simulink model "sampleModel2403_pp_difftest"  (R2018a)
settings: Solver=VariableStepAuto  StartTime=0.0  StopTime=10.0  RelTol=1e-3
undefined symbols (not defined in the file): DiscIntNeverNeededParam, sigbuilder_block
libraries: simulink x128
(part 1 of 3)
settings Model: Creator=cyfuzz  LastModifiedBy=ishaf
settings CodeAppCC: StateflowObjectComments=on

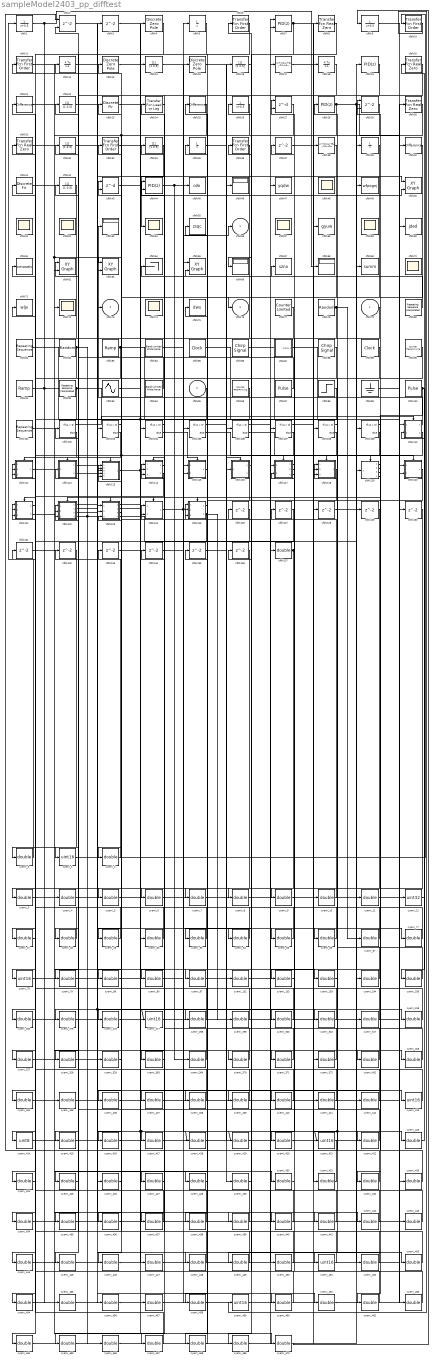
== system sampleModel2403_pp_difftest ==
  cfblk79 : Inport
  cfblk95 : Inport  Port=2
  cfblk1 : DiscreteTransferFcn  SampleTime=1
  cfblk{6,10..11,33,36} (5 alike) : simulink/Discrete/Transfer Fcn First Order  PoleZ=0.95  ICPrevOutput=0.0  DoSatur=off
      settings: SourceProductName=Simulink
  cfblk100 : DiscretePulseGenerator  PulseType=Time based  Period=10  PulseWidth=5
  cfblk101 : simulink/Sources/Repeating Sequence  rep_seq_t=[0 2]  rep_seq_y=[0 2]
  cfblk{102..109} (8 alike) : If  SampleTime=1
  cfblk110 : Subsystem  TreatAsAtomicUnit=on
  cfblk111 : Subsystem  TreatAsAtomicUnit=on
  cfblk112 : Subsystem  TreatAsAtomicUnit=on
  cfblk113 : Subsystem  TreatAsAtomicUnit=on
  cfblk114 : Subsystem  TreatAsAtomicUnit=on
  cfblk115 : Subsystem  TreatAsAtomicUnit=on
  cfblk116 : Subsystem  TreatAsAtomicUnit=on
  cfblk117 : Subsystem  TreatAsAtomicUnit=on
  cfblk118 : Subsystem  TreatAsAtomicUnit=on
  cfblk119 : Subsystem  TreatAsAtomicUnit=on
  cfblk12 : DiscreteIntegrator  OutDataTypeStr=double  ICPrevOutput=DiscIntNeverNeededParam  ICPrevScaledInput=DiscIntNeverNeededParam
  cfblk120 : Subsystem  TreatAsAtomicUnit=on
  cfblk121 : Subsystem  TreatAsAtomicUnit=on
  cfblk122 : Subsystem  TreatAsAtomicUnit=on
  cfblk123 : Subsystem  TreatAsAtomicUnit=on
  cfblk124 : Subsystem  TreatAsAtomicUnit=on
  cfblk125 : Subsystem  TreatAsAtomicUnit=on
  cfblk{3,37,126..136} (13 alike) : Delay  SampleTime=1
  cfblk13 : DiscreteZeroPole  Poles=[0 0.5]  Gain=1
  cfblk137 : DataTypeConversion  OutDataTypeStr=double
  cfblk{14,16,22,32,34,42} (6 alike) : DiscreteFilter  SampleTime=1
  cfblk15 : DiscreteZeroPole  Poles=[0 0.5]  Gain=1
  cfblk17 : DiscreteStateSpace
  cfblk18 : DiscreteIntegrator  OutDataTypeStr=double  ICPrevOutput=DiscIntNeverNeededParam  ICPrevScaledInput=DiscIntNeverNeededParam
  cfblk19 : simulink/Continuous/PID Controller  Controller=PID  TimeDomain=Discrete-time  SampleTime=1  IntegratorMethod=Forward Euler  FilterMethod=Forward Euler  Form=Parallel  UseFilter=on  ControllerParametersSource=internal  P=1  I=1  D=0  N=100  InitialConditionSource=internal  InitialConditionForIntegrator=0  InitialConditionForFilter=0  ExternalReset=none  LimitOutput=off  UpperSaturationLimit=inf  LowerSaturationLimit=-inf  LinearizeAsGain=off  AntiWindupMode=none  Kb=1  TrackingMode=off  Kt=1  PParamMin=[]  PParamMax=[]  IParamMin=[]  IParamMax=[]  DParamMin=[]  DParamMax=[]  NParamMin=[]  NParamMax=[]  KbParamMin=[]  KbParamMax=[]  KtParamMin=[]  KtParamMax=[]  POutMin=[]  POutMax=[]  IOutMin=[]  IOutMax=[]  DOutMin=[]  DOutMax=[]  NOutMin=[]  NOutMax=[]  KbOutMin=[]  KbOutMax=[]  KtOutMin=[]  KtOutMax=[]  IntegratorOutMin=[]  IntegratorOutMax=[]  FilterOutMin=[]  FilterOutMax=[]  SumOutMin=[]  SumOutMax=[]  SumI1OutMin=[]  SumI1OutMax=[]  SumI2OutMin=[]  SumI2OutMax=[]  SumI3OutMin=[]  SumI3OutMax=[]  SumDOutMin=[]  SumDOutMax=[]  SaturationOutMin=[]  SaturationOutMax=[]  IntegratorContinuousStateAttributes=''  IntegratorStateMustResolveToSignalObject=off  IntegratorRTWStateStorageClass=Auto  FilterContinuousStateAttributes=''  FilterStateMustResolveToSignalObject=off  FilterRTWStateStorageClass=Auto  DifferentiatorICPrevScaledInput=0  DifferentiatorOutMin=[]  DifferentiatorOutMax=[]  FilterDiffOutCoefMin=[]  FilterDiffOutCoefMax=[]  SumDenOutMin=[]  SumDenOutMax=[]  SumNumOutMin=[]  SumNumOutMax=[]  ReciprocalOutMin=[]  ReciprocalOutMax=[]  DivideOutMin=[]  DivideOutMax=[]  TunerSelectOption=Transfer Function Based (PID Tuner App)
  cfblk2 : Delay  ShowEnablePort=on  SampleTime=1
      settings: InputPortMap=u0,e6
  cfblk{8,20,30..31} (4 alike) : simulink/Discrete/Transfer Fcn Real Zero  ZeroZ=0.75  ICPrevInput=0.0  DoSatur=off
      settings: SourceProductName=Simulink  SourceProductBaseCode=SL
  cfblk21 : simulink/Discrete/Difference  ICPrevInput=0.0  OutMin=[]  OutMax=[]  OutDataTypeStr=double  OutputDataTypeScalingMode=double  OutDataType=fixdt(1, 16)  OutScaling=2^-10  DoSatur=off
  cfblk23 : DiscreteFir  SampleTime=1
  cfblk24 : simulink/Discrete/Transfer Fcn Lead or Lag  PoleZ=0.95  ZeroZ=0.75  ICPrevOutput=0.0  ICPrevInput=0.0  DoSatur=off
      settings: SourceProductName=Simulink  SourceProductBaseCode=SL
  cfblk25 : simulink/Discrete/Difference  ICPrevInput=0.0  OutMin=[]  OutMax=[]  OutDataTypeStr=double  OutputDataTypeScalingMode=double  OutDataType=fixdt(1, 16)  OutScaling=2^-10  DoSatur=off
  cfblk26 : DiscreteTransferFcn  SampleTime=1
  cfblk27 : Delay  DelayLengthSource=Input port  SampleTime=1
      settings: InputPortMap=u0,p1
  cfblk28 : simulink/Continuous/PID Controller  Controller=PID  TimeDomain=Discrete-time  SampleTime=1  IntegratorMethod=Forward Euler  FilterMethod=Forward Euler  Form=Parallel  UseFilter=on  ControllerParametersSource=internal  P=1  I=1  D=0  N=100  InitialConditionSource=internal  InitialConditionForIntegrator=0  InitialConditionForFilter=0  ExternalReset=none  LimitOutput=off  UpperSaturationLimit=inf  LowerSaturationLimit=-inf  LinearizeAsGain=off  AntiWindupMode=none  Kb=1  TrackingMode=off  Kt=1  PParamMin=[]  PParamMax=[]  IParamMin=[]  IParamMax=[]  DParamMin=[]  DParamMax=[]  NParamMin=[]  NParamMax=[]  KbParamMin=[]  KbParamMax=[]  KtParamMin=[]  KtParamMax=[]  POutMin=[]  POutMax=[]  IOutMin=[]  IOutMax=[]  DOutMin=[]  DOutMax=[]  NOutMin=[]  NOutMax=[]  KbOutMin=[]  KbOutMax=[]  KtOutMin=[]  KtOutMax=[]  IntegratorOutMin=[]  IntegratorOutMax=[]  FilterOutMin=[]  FilterOutMax=[]  SumOutMin=[]  SumOutMax=[]  SumI1OutMin=[]  SumI1OutMax=[]  SumI2OutMin=[]  SumI2OutMax=[]  SumI3OutMin=[]  SumI3OutMax=[]  SumDOutMin=[]  SumDOutMax=[]  SaturationOutMin=[]  SaturationOutMax=[]  IntegratorContinuousStateAttributes=''  IntegratorStateMustResolveToSignalObject=off  IntegratorRTWStateStorageClass=Auto  FilterContinuousStateAttributes=''  FilterStateMustResolveToSignalObject=off  FilterRTWStateStorageClass=Auto  DifferentiatorICPrevScaledInput=0  DifferentiatorOutMin=[]  DifferentiatorOutMax=[]  FilterDiffOutCoefMin=[]  FilterDiffOutCoefMax=[]  SumDenOutMin=[]  SumDenOutMax=[]  SumNumOutMin=[]  SumNumOutMax=[]  ReciprocalOutMin=[]  ReciprocalOutMax=[]  DivideOutMin=[]  DivideOutMax=[]  TunerSelectOption=Transfer Function Based (PID Tuner App)
  cfblk29 : Delay  ShowEnablePort=on  SampleTime=1
      settings: InputPortMap=u0,e6
  cfblk35 : UnitDelay
  cfblk38 : DiscreteStateSpace
  cfblk39 : UnitDelay
  cfblk4 : DiscreteZeroPole  Poles=[0 0.5]  Gain=1
  cfblk40 : simulink/Discrete/Difference  ICPrevInput=0.0  OutMin=[]  OutMax=[]  OutDataTypeStr=double  OutputDataTypeScalingMode=double  OutDataType=fixdt(1, 16)  OutScaling=2^-10  DoSatur=off
  cfblk41 : DiscreteFir  SampleTime=1
  cfblk43 : Delay  DelayLengthSource=Input port  SampleTime=1
      settings: InputPortMap=u0,p1
  cfblk44 : simulink/Continuous/PID Controller (2DOF)  Controller=PID  TimeDomain=Discrete-time  SampleTime=1  IntegratorMethod=Forward Euler  FilterMethod=Forward Euler  Form=Parallel  UseFilter=on  ControllerParametersSource=internal  P=1  I=1  D=0  N=100  b=1  c=1  InitialConditionSource=internal  InitialConditionForIntegrator=0  InitialConditionForFilter=0  ExternalReset=none  LimitOutput=off  UpperSaturationLimit=inf  LowerSaturationLimit=-inf  LinearizeAsGain=off  AntiWindupMode=none  Kb=1  TrackingMode=off  Kt=1  PParamMin=[]  PParamMax=[]  IParamMin=[]  IParamMax=[]  DParamMin=[]  DParamMax=[]  NParamMin=[]  NParamMax=[]  bParamMin=[]  bParamMax=[]  cParamMin=[]  cParamMax=[]  KbParamMin=[]  KbParamMax=[]  KtParamMin=[]  KtParamMax=[]  POutMin=[]  POutMax=[]  IOutMin=[]  IOutMax=[]  DOutMin=[]  DOutMax=[]  NOutMin=[]  NOutMax=[]  bOutMin=[]  bOutMax=[]  cOutMin=[]  cOutMax=[]  KbOutMin=[]  KbOutMax=[]  KtOutMin=[]  KtOutMax=[]  IntegratorOutMin=[]  IntegratorOutMax=[]  FilterOutMin=[]  FilterOutMax=[]  SumOutMin=[]  SumOutMax=[]  Sum1OutMin=[]  Sum1OutMax=[]  Sum2OutMin=[]  Sum2OutMax=[]  Sum3OutMin=[]  Sum3OutMax=[]  SumI1OutMin=[]  SumI1OutMax=[]  SumI2OutMin=[]  SumI2OutMax=[]  SumI3OutMin=[]  SumI3OutMax=[]  SumDOutMin=[]  SumDOutMax=[]  SaturationOutMin=[]  SaturationOutMax=[]  IntegratorContinuousStateAttributes=''  IntegratorStateMustResolveToSignalObject=off  IntegratorRTWStateStorageClass=Auto  FilterContinuousStateAttributes=''  FilterStateMustResolveToSignalObject=off  FilterRTWStateStorageClass=Auto  DifferentiatorICPrevScaledInput=0  DifferentiatorOutMin=[]  DifferentiatorOutMax=[]  FilterDiffOutCoefMin=[]  FilterDiffOutCoefMax=[]  SumDenOutMin=[]  SumDenOutMax=[]  SumNumOutMin=[]  SumNumOutMax=[]  ReciprocalOutMin=[]  ReciprocalOutMax=[]  DivideOutMin=[]  DivideOutMax=[]  TunerSelectOption=Transfer Function Based (PID Tuner App)
  cfblk45 : ToFile  Filename=oilo  SaveFormat=Timeseries
  cfblk{46,53,66,68} (4 alike) : Display
  cfblk47 : ToFile  Filename=yqdw  SaveFormat=Timeseries
  cfblk{48,51..52,54,57,59,70,72,74} (9 alike) : Scope
      cfblk48 settings: Floating=on
      cfblk51 settings: Floating=on
      cfblk52 settings: Floating=on
      cfblk57 settings: Floating=on
      cfblk59 settings: Floating=on
      cfblk70 settings: Floating=on
      cfblk74 settings: Floating=on
  cfblk49 : ToWorkspace  VariableName=wfpognj  SaveFormat=Timeseries  SampleTime=-1
  cfblk5 : UnitDelay
  cfblk{50,62..63,65} (4 alike) : simulink/Sinks/XY Graph  xmin=-1  xmax=1  ymin=-1  ymax=1  st=-1
  cfblk55 : ToFile  Filename=zsqc  SaveFormat=Timeseries
  cfblk58 : ToFile  Filename=gyuw  SaveFormat=Timeseries
  cfblk60 : ToFile  Filename=jded  SaveFormat=Timeseries
  cfblk61 : ToWorkspace  VariableName=xmoseic  SaveFormat=Timeseries  SampleTime=-1
  cfblk64 : Terminator
  cfblk67 : ToFile  Filename=szno  SaveFormat=Timeseries
  cfblk69 : ToFile  Filename=summ  SaveFormat=Timeseries
  cfblk7 : simulink/Continuous/PID Controller (2DOF)  Controller=PID  TimeDomain=Discrete-time  SampleTime=1  IntegratorMethod=Forward Euler  FilterMethod=Forward Euler  Form=Parallel  UseFilter=on  ControllerParametersSource=internal  P=1  I=1  D=0  N=100  b=1  c=1  InitialConditionSource=internal  InitialConditionForIntegrator=0  InitialConditionForFilter=0  ExternalReset=none  LimitOutput=off  UpperSaturationLimit=inf  LowerSaturationLimit=-inf  LinearizeAsGain=off  AntiWindupMode=none  Kb=1  TrackingMode=off  Kt=1  PParamMin=[]  PParamMax=[]  IParamMin=[]  IParamMax=[]  DParamMin=[]  DParamMax=[]  NParamMin=[]  NParamMax=[]  bParamMin=[]  bParamMax=[]  cParamMin=[]  cParamMax=[]  KbParamMin=[]  KbParamMax=[]  KtParamMin=[]  KtParamMax=[]  POutMin=[]  POutMax=[]  IOutMin=[]  IOutMax=[]  DOutMin=[]  DOutMax=[]  NOutMin=[]  NOutMax=[]  bOutMin=[]  bOutMax=[]  cOutMin=[]  cOutMax=[]  KbOutMin=[]  KbOutMax=[]  KtOutMin=[]  KtOutMax=[]  IntegratorOutMin=[]  IntegratorOutMax=[]  FilterOutMin=[]  FilterOutMax=[]  SumOutMin=[]  SumOutMax=[]  Sum1OutMin=[]  Sum1OutMax=[]  Sum2OutMin=[]  Sum2OutMax=[]  Sum3OutMin=[]  Sum3OutMax=[]  SumI1OutMin=[]  SumI1OutMax=[]  SumI2OutMin=[]  SumI2OutMax=[]  SumI3OutMin=[]  SumI3OutMax=[]  SumDOutMin=[]  SumDOutMax=[]  SaturationOutMin=[]  SaturationOutMax=[]  IntegratorContinuousStateAttributes=''  IntegratorStateMustResolveToSignalObject=off  IntegratorRTWStateStorageClass=Auto  FilterContinuousStateAttributes=''  FilterStateMustResolveToSignalObject=off  FilterRTWStateStorageClass=Auto  DifferentiatorICPrevScaledInput=0  DifferentiatorOutMin=[]  DifferentiatorOutMax=[]  FilterDiffOutCoefMin=[]  FilterDiffOutCoefMax=[]  SumDenOutMin=[]  SumDenOutMax=[]  SumNumOutMin=[]  SumNumOutMax=[]  ReciprocalOutMin=[]  ReciprocalOutMax=[]  DivideOutMin=[]  DivideOutMax=[]  TunerSelectOption=Transfer Function Based (PID Tuner App)
  cfblk71 : ToFile  Filename=wljx  SaveFormat=Timeseries
  cfblk75 : ToFile  Filename=itws  SaveFormat=Timeseries
  cfblk77 : simulink/Sources/Counter Limited  uplimit=7  tsamp=-1
  cfblk78 : UniformRandomNumber  SampleTime=0.1
  cfblk80 : simulink/Sources/Repeating Sequence Interpolated  OutValues=[3 1 4 2 1].'  TimeValues=[0 0.1 0.5 0.6 1].'  LookUpMeth=Interpolation-Use End Values  tsamp=0.01  OutMin=[]  OutMax=[]  OutDataTypeStr=double  OutputDataTypeScalingMode=double  OutDataType=fixdt(0,8)  OutScaling=2^-10
  cfblk81 : simulink/Sources/Repeating Sequence  rep_seq_t=[0 2]  rep_seq_y=[0 2]
  cfblk82 : UniformRandomNumber  SampleTime=0.1
  cfblk83 : simulink/Sources/Ramp  slope=1  start=0  InitialOutput=0
  cfblk84 : simulink/Sources/Band-Limited White Noise  Cov=[0.1]  Ts=0.1  seed=[23341]
  cfblk85 : DigitalClock
  cfblk86 : simulink/Sources/Chirp Signal  f1=0.1  T=100  f2=1
  cfblk87 : Subsystem  Tag=STV Subsys  LoadFcn=sigbuilder_block('load');  StartFcn=sigbuilder_block('start');  StopFcn=sigbuilder_block('stop');  ClipboardFcn=sigbuilder_block('clipboard');  mask(Sigbuilder block){tuvar=[0:10]}
      mask help: Simulink:masks:SigbuilderBlock_MD
      mask init:
      | if ~strcmp(get_param(bdroot(gcbh),'SimulationStatus'),'stopped') tuvar = sigbuilder_block('maskInit'); end
      settings: CopyFcn=sigbuilder_block('copy');  DeleteFcn=sigbuilder_block('delete');  ModelCloseFcn=sigbuilder_block('modelClose');  PreSaveFcn=sigbuilder_block('preSave');  PauseFcn=sigbuilder_block('pause');  ContinueFcn=sigbuilder_block('continue');  NameChangeFcn=sigbuilder_block('namechange');  OpenFcn=sigbuilder_block('open',[437.6 199.2 550.4 400 ]);  CloseFcn=sigbuilder_block('close');
      mask Display: plot(0, 0, 100, 100,[2, 2, 32, 32, 2], [68, 8, 8, 68, 68],[32, 2], [38, 38], [32, 19, 2],[53, 60, 44], [32, 17, 17, 2],[16, 16, 31, 31]);txt = getActiveGroup(gcbh);text(2, 100, txt,'verticalAlignment', 'top');
  cfblk88 : simulink/Sources/Chirp Signal  f1=0.1  T=100  f2=1
  cfblk89 : DigitalClock
  cfblk9 : DiscreteTransferFcn  SampleTime=1
  cfblk90 : simulink/Sources/Counter Free-Running  NumBits=16  tsamp=-1
  cfblk91 : simulink/Sources/Ramp  slope=1  start=0  InitialOutput=0
  cfblk92 : simulink/Sources/Repeating Sequence Interpolated  OutValues=[3 1 4 2 1].'  TimeValues=[0 0.1 0.5 0.6 1].'  LookUpMeth=Interpolation-Use End Values  tsamp=0.01  OutMin=[]  OutMax=[]  OutDataTypeStr=double  OutputDataTypeScalingMode=double  OutDataType=fixdt(0,8)  OutScaling=2^-10
  cfblk93 : Sin  SampleTime=0
  cfblk94 : simulink/Sources/Band-Limited White Noise  Cov=[0.1]  Ts=0.1  seed=[23341]
  cfblk96 : simulink/Sources/Counter Free-Running  NumBits=16  tsamp=-1
  cfblk97 : DiscretePulseGenerator  PulseType=Time based  Period=10  PulseWidth=5
  cfblk98 : Step  After=21  SampleTime=0
  cfblk99 : Ground
  cyemi_{0,2..11,47..49,53,63..67,77,79,89..90,97,132..133,193..195,262,275..276,298..300,316..318,327..329,363..364,370..372,402..412,415..420,422..450,452..458,460..470} (111 alike) : DataTypeConversion  OutDataTypeStr=double
  cyemi_{1,78,277,413,421,451,459} (7 alike) : DataTypeConversion  OutDataTypeStr=uint16
  cyemi_12 : DataTypeConversion  OutDataTypeStr=uint32
  cyemi_414 : DataTypeConversion  OutDataTypeStr=uint8
  cfblk56 : Outport
  cfblk73 : Outport  Port=2
  cfblk76 : Outport  Port=3
  wires:
  cfblk110/1(cfblk2) -> cfblk53/1
  cfblk80/1 -> cfblk64/1
  cfblk11/1 -> cfblk72/1, cfblk63/2
  cfblk1/1 -> cfblk68/1, cyemi_4/1
  cfblk32/1 -> cyemi_417/1, cyemi_418/1
  cfblk84/1 -> cfblk65/1
  cfblk91/1 -> cyemi_450/1, cyemi_455/1
  cfblk13/1 -> cyemi_419/1, cyemi_448/1
  cfblk34/1 -> cfblk54/1
  cfblk83/1 -> cyemi_47/1, cyemi_431/1
  cfblk82/1 -> cyemi_464/1, cyemi_466/1
  cfblk90/1 -> cyemi_421/1, cyemi_451/1
  cfblk35/1 -> cfblk46/1
  cfblk97/1 -> cfblk62/1
  cfblk78/1 -> cyemi_67/1, cyemi_469/1
  cfblk100/1 -> cyemi_195/1, cyemi_432/1
  cfblk125/2(cfblk13) -> cyemi_6/1, cyemi_299/1
  cfblk81/1 -> cyemi_372/1, cyemi_447/1
  cfblk124/1(cfblk2) -> cfblk56/1, cyemi_371/1
  cfblk94/1 -> cfblk73/1
  cfblk22/1 -> cfblk50/1
  cfblk25/1 -> cfblk62/2
  cfblk8/1 -> cfblk76/1
  cfblk92/1 -> cyemi_317/1, cyemi_434/1
  cfblk28/1 -> cfblk63/1, cyemi_48/1, cyemi_423/1, cyemi_433/1
  cfblk7/1 -> cfblk66/1, cyemi_402/1
  cfblk110/2(cfblk10) -> cyemi_49/1, cyemi_328/1
  cfblk117/3(cfblk13) -> cfblk65/2
  cfblk44/1 -> cyemi_364/1, cyemi_422/1
  cfblk2/1 -> cyemi_277/1, cyemi_413/1
  cfblk122/4(cfblk14) -> cyemi_66/1, cyemi_329/1
  cfblk113/1(cfblk2) -> cfblk50/2, cyemi_410/1
  cfblk102/1 -> cfblk110/Action
  cfblk102/2 -> cfblk111/Action
  cfblk103/1 -> cfblk112/Action
  cfblk103/2 -> cfblk113/Action
  cfblk104/1 -> cfblk114/Action
  cfblk104/2 -> cfblk115/Action
  cfblk105/1 -> cfblk116/Action
  cfblk105/2 -> cfblk117/Action
  cfblk106/1 -> cfblk118/Action
  cfblk106/2 -> cfblk119/Action
  cfblk107/1 -> cfblk120/Action
  cfblk107/2 -> cfblk121/Action
  cfblk108/1 -> cfblk122/Action
  cfblk108/2 -> cfblk123/Action
  cfblk109/1 -> cfblk124/Action
  cfblk109/2 -> cfblk125/Action
  cfblk137/1 -> cyemi_300/1, cyemi_406/1
  cyemi_0/1 -> cfblk1/1
  cfblk126/1 -> cyemi_0/1
  cyemi_1/1 -> cfblk10/1
  cfblk96/1 -> cyemi_1/1
  cyemi_2/1 -> cfblk102/1
  cfblk40/1 -> cyemi_2/1
  cyemi_3/1 -> cfblk103/1
  cfblk95/1 -> cyemi_3/1
  cyemi_4/1 -> cfblk104/1
  cyemi_5/1 -> cfblk105/1
  cfblk88/1 -> cyemi_5/1
  cyemi_6/1 -> cfblk106/1
  cyemi_7/1 -> cfblk107/1
  cfblk125/1(cfblk2) -> cyemi_7/1
  cyemi_8/1 -> cfblk108/1
  cfblk38/1 -> cyemi_8/1
  cyemi_9/1 -> cfblk109/1
  cfblk129/1 -> cyemi_9/1
  cyemi_10/1 -> cfblk11/1
  cfblk37/1 -> cyemi_10/1
  cyemi_11/1 -> cfblk110/1(cfblk1)
  cfblk86/1 -> cyemi_11/1
  cyemi_12/1 -> cfblk110/2(cfblk9)
  cfblk99/1 -> cyemi_12/1
  cyemi_47/1 -> cfblk111/1(cfblk1)
  cyemi_48/1 -> cfblk111/2(cfblk6)
  cyemi_49/1 -> cfblk111/3(cfblk7)
  cyemi_53/1 -> cfblk112/1(cfblk1)
  cfblk93/1 -> cyemi_53/1
  cyemi_63/1 -> cfblk113/1(cfblk1)
  cfblk116/1(cfblk2) -> cyemi_63/1
  cyemi_64/1 -> cfblk113/2(cfblk12)
  cfblk16/1 -> cyemi_64/1
  cyemi_65/1 -> cfblk113/3(cfblk13)
  cfblk23/1 -> cyemi_65/1
  cyemi_66/1 -> cfblk113/4(cfblk14)
  cyemi_67/1 -> cfblk113/5(cfblk15)
  cyemi_77/1 -> cfblk114/1(cfblk1)
  cfblk14/1 -> cyemi_77/1
  cyemi_78/1 -> cfblk114/2(cfblk8)
  cfblk136/1 -> cyemi_78/1
  cyemi_79/1 -> cfblk114/3(cfblk9)
  cfblk127/1 -> cyemi_79/1
  cyemi_89/1 -> cfblk115/1(cfblk1)
  cfblk39/1 -> cyemi_89/1
  cyemi_90/1 -> cfblk115/2(cfblk8)
  cfblk130/1 -> cyemi_90/1
  cyemi_97/1 -> cfblk116/1(cfblk1)
  cfblk41/1 -> cyemi_97/1
  cyemi_132/1 -> cfblk117/1(cfblk1)
  cfblk135/1 -> cyemi_132/1
  cyemi_133/1 -> cfblk117/2(cfblk11)
  cfblk119/3(cfblk13) -> cyemi_133/1
  cyemi_193/1 -> cfblk118/1(cfblk1)
  cfblk134/1 -> cyemi_193/1
  cyemi_194/1 -> cfblk118/2(cfblk15)
  cfblk87/1(Signal 1) -> cyemi_194/1
  cyemi_195/1 -> cfblk118/3(cfblk16)
  cyemi_262/1 -> cfblk119/1(cfblk1)
  cfblk36/1 -> cyemi_262/1
  cyemi_275/1 -> cfblk12/1
  cfblk117/2(cfblk12) -> cyemi_275/1
  cyemi_276/1 -> cfblk120/1(cfblk1)
  cfblk116/2(cfblk15) -> cyemi_276/1
  cyemi_277/1 -> cfblk120/2(cfblk16)
  cyemi_298/1 -> cfblk121/1(cfblk1)
  cfblk118/1(cfblk2) -> cyemi_298/1
  cyemi_299/1 -> cfblk121/2(cfblk15)
  cyemi_300/1 -> cfblk121/3(cfblk16)
  cyemi_316/1 -> cfblk122/1(cfblk1)
  cfblk33/1 -> cyemi_316/1
  cyemi_317/1 -> cfblk122/2(cfblk10)
  cyemi_318/1 -> cfblk122/3(cfblk11)
  cfblk133/1 -> cyemi_318/1
  cyemi_327/1 -> cfblk123/1(cfblk1)
  cfblk132/1 -> cyemi_327/1
  cyemi_328/1 -> cfblk123/2(cfblk12)
  cyemi_329/1 -> cfblk123/3(cfblk13)
  cyemi_363/1 -> cfblk124/1(cfblk1)
  cfblk19/1 -> cyemi_363/1
  cyemi_364/1 -> cfblk124/2(cfblk7)
  cyemi_370/1 -> cfblk125/1(cfblk1)
  cfblk131/1 -> cyemi_370/1
  cyemi_371/1 -> cfblk125/2(cfblk11)
  cyemi_372/1 -> cfblk125/3(cfblk12)
  cyemi_402/1 -> cfblk126/1
  cyemi_403/1 -> cfblk127/1
  cfblk122/1(cfblk2) -> cyemi_403/1
  cyemi_404/1 -> cfblk128/1
  cfblk121/1(cfblk2) -> cyemi_404/1
  cyemi_405/1 -> cfblk129/1
  cfblk21/1 -> cyemi_405/1
  cyemi_406/1 -> cfblk13/1
  cyemi_407/1 -> cfblk130/1
  cfblk119/2(cfblk12) -> cyemi_407/1
  cyemi_408/1 -> cfblk131/1
  cfblk115/1(cfblk2) -> cyemi_408/1
  cyemi_409/1 -> cfblk132/1
  cfblk117/1(cfblk2) -> cyemi_409/1
  cyemi_410/1 -> cfblk133/1
  cyemi_411/1 -> cfblk134/1
  cfblk17/1 -> cyemi_411/1
  cyemi_412/1 -> cfblk135/1
  cfblk123/4(cfblk16) -> cyemi_412/1
  cyemi_413/1 -> cfblk136/1
  cyemi_414/1 -> cfblk137/1
  cfblk77/1 -> cyemi_414/1
  cyemi_415/1 -> cfblk14/1
  cfblk18/1 -> cyemi_415/1
  cyemi_416/1 -> cfblk15/1
  cfblk30/1 -> cyemi_416/1
  cyemi_417/1 -> cfblk16/1
  cyemi_418/1 -> cfblk17/1
  cyemi_419/1 -> cfblk18/1
  cyemi_420/1 -> cfblk19/1
  cfblk79/1 -> cyemi_420/1
  cyemi_421/1 -> cfblk2/1
  cyemi_422/1 -> cfblk2/2
  cyemi_423/1 -> cfblk20/1
  cyemi_424/1 -> cfblk21/1
  cfblk4/1 -> cyemi_424/1
  cyemi_425/1 -> cfblk22/1
  cfblk120/1(cfblk2) -> cyemi_425/1
  cyemi_426/1 -> cfblk23/1
  cfblk12/1 -> cyemi_426/1
  cyemi_427/1 -> cfblk24/1
  cfblk29/1 -> cyemi_427/1
  cyemi_428/1 -> cfblk25/1
  cfblk6/1 -> cyemi_428/1
  cyemi_429/1 -> cfblk26/1
  cfblk15/1 -> cyemi_429/1
  cyemi_430/1 -> cfblk27/1
  cfblk121/2(cfblk17) -> cyemi_430/1
  cyemi_431/1 -> cfblk27/2
  cyemi_432/1 -> cfblk28/1
  cyemi_433/1 -> cfblk29/1
  cyemi_434/1 -> cfblk29/2
  cyemi_435/1 -> cfblk3/1
  cfblk5/1 -> cyemi_435/1
  cyemi_436/1 -> cfblk30/1
  cfblk123/3(cfblk15) -> cyemi_436/1
  cyemi_437/1 -> cfblk31/1
  cfblk24/1 -> cyemi_437/1
  cyemi_438/1 -> cfblk32/1
  cfblk26/1 -> cyemi_438/1
  cyemi_439/1 -> cfblk33/1
  cfblk111/1(cfblk2) -> cyemi_439/1
  cyemi_440/1 -> cfblk34/1
  cfblk112/2(cfblk9) -> cyemi_440/1
  cyemi_441/1 -> cfblk35/1
  cfblk31/1 -> cyemi_441/1
  cyemi_442/1 -> cfblk36/1
  cfblk43/1 -> cyemi_442/1
  cyemi_443/1 -> cfblk37/1
  cfblk85/1 -> cyemi_443/1
  cyemi_444/1 -> cfblk38/1
  cfblk114/2(cfblk10) -> cyemi_444/1
  cyemi_445/1 -> cfblk39/1
  cfblk89/1 -> cyemi_445/1
  cyemi_446/1 -> cfblk4/1
  cfblk27/1 -> cyemi_446/1
  cyemi_447/1 -> cfblk40/1
  cyemi_448/1 -> cfblk41/1
  cyemi_449/1 -> cfblk42/1
  cfblk119/1(cfblk2) -> cyemi_449/1
  cyemi_450/1 -> cfblk43/1
  cyemi_451/1 -> cfblk43/2
  cyemi_452/1 -> cfblk44/1
  cfblk128/1 -> cyemi_452/1
  cyemi_453/1 -> cfblk44/2
  cfblk122/3(cfblk13) -> cyemi_453/1
  cyemi_454/1 -> cfblk45/1
  cfblk42/1 -> cyemi_454/1
  cyemi_455/1 -> cfblk47/1
  cyemi_456/1 -> cfblk49/1
  cfblk112/1(cfblk2) -> cyemi_456/1
  cyemi_457/1 -> cfblk5/1
  cfblk123/2(cfblk14) -> cyemi_457/1
  cyemi_458/1 -> cfblk55/1
  cfblk20/1 -> cyemi_458/1
  cyemi_459/1 -> cfblk58/1
  cfblk10/1 -> cyemi_459/1
  cyemi_460/1 -> cfblk6/1
  cfblk122/2(cfblk12) -> cyemi_460/1
  cyemi_461/1 -> cfblk60/1
  cfblk123/1(cfblk2) -> cyemi_461/1
  cyemi_462/1 -> cfblk61/1
  cfblk119/4(cfblk14) -> cyemi_462/1
  cyemi_463/1 -> cfblk67/1
  cfblk9/1 -> cyemi_463/1
  cyemi_464/1 -> cfblk69/1
  cyemi_465/1 -> cfblk7/1
  cfblk114/1(cfblk2) -> cyemi_465/1
  cyemi_466/1 -> cfblk7/2
  cyemi_467/1 -> cfblk71/1
  cfblk101/1 -> cyemi_467/1
  cyemi_468/1 -> cfblk75/1
  cfblk98/1 -> cyemi_468/1
  cyemi_469/1 -> cfblk8/1
  cyemi_470/1 -> cfblk9/1
  cfblk3/1 -> cyemi_470/1

== system sampleModel2403_pp_difftest/cfblk110 ==
  cfblk1 : Inport
  cfblk9 : Inport  Port=2
  Action Port : ActionPort  ActionType=then
  cfblk11 : Subsystem  TreatAsAtomicUnit=on
  cfblk12 : Subsystem  TreatAsAtomicUnit=on
  cfblk13 : Delay
  cfblk14 : Delay
  cfblk3 : simulink/Discrete/Tapped Delay  vinit=0.0  samptime=-1  NumDelays=1  DelayOrder=Oldest  includeCurrent=off
  cfblk4 : Delay
  cfblk5 : DiscreteTransferFcn
  cfblk6 : simulink/Discrete/Transfer Fcn Real Zero  ZeroZ=0.75  ICPrevInput=0.0  DoSatur=off
      settings: SourceProductName=Simulink  SourceProductBaseCode=SL
  cfblk7 : DiscreteFir
  cfblk8 : If  SampleTime=1
  cyemi_13 : DataTypeConversion  OutDataTypeStr=uint32
  cyemi_{14,34,40..46} (9 alike) : DataTypeConversion  OutDataTypeStr=double
  cyemi_33 : DataTypeConversion  OutDataTypeStr=uint32
  cyemi_39 : DataTypeConversion  OutDataTypeStr=uint32
  cfblk2 : Outport
  cfblk10 : Outport  Port=2
  wires:
  cfblk12/1(cfblk2) -> cfblk2/1
  cfblk4/1 -> cyemi_14/1, cyemi_41/1
  cfblk5/1 -> cfblk10/1
  cfblk8/1 -> cfblk11/Action
  cfblk8/2 -> cfblk12/Action
  cyemi_13/1 -> cfblk11/1(cfblk1)
  cfblk9/1 -> cyemi_13/1
  cyemi_14/1 -> cfblk11/2(cfblk15)
  cyemi_33/1 -> cfblk12/1(cfblk1)
  cfblk13/1 -> cyemi_33/1
  cyemi_34/1 -> cfblk12/2(cfblk7)
  cfblk6/1 -> cyemi_34/1
  cyemi_39/1 -> cfblk13/1
  cfblk11/1(cfblk2) -> cyemi_39/1
  cyemi_40/1 -> cfblk14/1
  cfblk12/3(cfblk9) -> cyemi_40/1
  cyemi_41/1 -> cfblk3/1
  cyemi_42/1 -> cfblk4/1
  cfblk1/1 -> cyemi_42/1
  cyemi_43/1 -> cfblk5/1
  cfblk12/2(cfblk8) -> cyemi_43/1
  cyemi_44/1 -> cfblk6/1
  cfblk7/1 -> cyemi_44/1
  cyemi_45/1 -> cfblk7/1
  cfblk3/1 -> cyemi_45/1
  cyemi_46/1 -> cfblk8/1
  cfblk14/1 -> cyemi_46/1

== system sampleModel2403_pp_difftest/cfblk111 ==
  cfblk1 : Inport
  cfblk6 : Inport  Port=2
  cfblk7 : Inport  Port=3
  Action Port : ActionPort  ActionType=else
  cfblk3 : Delay
  cfblk4 : DiscreteTransferFcn
  cfblk5 : simulink/Discrete/Transfer Fcn Real Zero  ZeroZ=0.75  ICPrevInput=0.0  DoSatur=off
      settings: SourceProductName=Simulink  SourceProductBaseCode=SL
  cyemi_50 : DataTypeConversion  OutDataTypeStr=double
  cyemi_51 : DataTypeConversion  OutDataTypeStr=double
  cyemi_52 : DataTypeConversion  OutDataTypeStr=double
  cfblk2 : Outport
  wires:
  cfblk5/1 -> cfblk2/1
  cyemi_50/1 -> cfblk3/1
  cfblk7/1 -> cyemi_50/1
  cyemi_51/1 -> cfblk4/1
  cfblk3/1 -> cyemi_51/1
  cyemi_52/1 -> cfblk5/1
  cfblk1/1 -> cyemi_52/1

== system sampleModel2403_pp_difftest/cfblk112 ==
  cfblk1 : Inport
  Action Port : ActionPort  ActionType=then
  cfblk10 : Delay
  cfblk3 : DiscreteIntegrator  SampleTime=-1  OutDataTypeStr=double  ICPrevOutput=DiscIntNeverNeededParam  ICPrevScaledInput=DiscIntNeverNeededParam
  cfblk4 : Delay  DelayLengthSource=Input port
      settings: InputPortMap=u0,p1
  cfblk5 : simulink/Discrete/Transfer Fcn Real Zero  ZeroZ=0.75  ICPrevInput=0.0  DoSatur=off
      settings: SourceProductName=Simulink  SourceProductBaseCode=SL
  cfblk6 : Delay  ShowEnablePort=on
      settings: InputPortMap=u0,e6
  cfblk7 : simulink/Discrete/Transfer Fcn Real Zero  ZeroZ=0.75  ICPrevInput=0.0  DoSatur=off
      settings: SourceProductName=Simulink  SourceProductBaseCode=SL
  cfblk8 : DiscreteFilter
  cyemi_{54..62} (9 alike) : DataTypeConversion  OutDataTypeStr=double
  cfblk2 : Outport
  cfblk9 : Outport  Port=2
  wires:
  cfblk6/1 -> cyemi_55/1, cyemi_56/1
  cfblk7/1 -> cfblk9/1
  cfblk3/1 -> cyemi_57/1, cyemi_58/1
  cfblk1/1 -> cyemi_60/1, cyemi_62/1
  cfblk5/1 -> cfblk2/1
  cyemi_54/1 -> cfblk10/1
  cfblk4/1 -> cyemi_54/1
  cyemi_55/1 -> cfblk3/1
  cyemi_56/1 -> cfblk4/1
  cyemi_57/1 -> cfblk4/2
  cyemi_58/1 -> cfblk5/1
  cyemi_59/1 -> cfblk6/1
  cfblk10/1 -> cyemi_59/1
  cyemi_60/1 -> cfblk6/2
  cyemi_61/1 -> cfblk7/1
  cfblk8/1 -> cyemi_61/1
  cyemi_62/1 -> cfblk8/1

== system sampleModel2403_pp_difftest/cfblk113 ==
  cfblk1 : Inport
  cfblk12 : Inport  Port=2
  cfblk13 : Inport  Port=3
  cfblk14 : Inport  Port=4
  cfblk15 : Inport  Port=5
  Action Port : ActionPort  ActionType=else
  cfblk10 : DiscreteStateSpace  SampleTime=-1
  cfblk11 : UnitDelay  SampleTime=-1
  cfblk3 : simulink/Discrete/Transfer Fcn Real Zero  ZeroZ=0.75  ICPrevInput=0.0  DoSatur=off
      settings: SourceProductName=Simulink  SourceProductBaseCode=SL
  cfblk4 : simulink/Discrete/Tapped Delay  vinit=0.0  samptime=-1  NumDelays=1  DelayOrder=Oldest  includeCurrent=off
  cfblk5 : DiscreteTransferFcn
  cfblk6 : DiscreteIntegrator  SampleTime=-1  OutDataTypeStr=double  ICPrevOutput=DiscIntNeverNeededParam  ICPrevScaledInput=DiscIntNeverNeededParam
  cfblk7 : simulink/Discrete/Transfer Fcn Lead or Lag  PoleZ=0.95  ZeroZ=0.75  ICPrevOutput=0.0  ICPrevInput=0.0  DoSatur=off
      settings: SourceProductName=Simulink  SourceProductBaseCode=SL
  cfblk8 : simulink/Discrete/Transfer Fcn Lead or Lag  PoleZ=0.95  ZeroZ=0.75  ICPrevOutput=0.0  ICPrevInput=0.0  DoSatur=off
      settings: SourceProductName=Simulink  SourceProductBaseCode=SL
  cfblk9 : UnitDelay  SampleTime=-1
  cyemi_{68..76} (9 alike) : DataTypeConversion  OutDataTypeStr=double
  cfblk2 : Outport
  wires:
  cfblk14/1 -> cfblk2/1
  cyemi_68/1 -> cfblk10/1
  cfblk1/1 -> cyemi_68/1
  cyemi_69/1 -> cfblk11/1
  cfblk5/1 -> cyemi_69/1
  cyemi_70/1 -> cfblk3/1
  cfblk13/1 -> cyemi_70/1
  cyemi_71/1 -> cfblk4/1
  cfblk9/1 -> cyemi_71/1
  cyemi_72/1 -> cfblk5/1
  cfblk10/1 -> cyemi_72/1
  cyemi_73/1 -> cfblk6/1
  cfblk11/1 -> cyemi_73/1
  cyemi_74/1 -> cfblk7/1
  cfblk8/1 -> cyemi_74/1
  cyemi_75/1 -> cfblk8/1
  cfblk12/1 -> cyemi_75/1
  cyemi_76/1 -> cfblk9/1
  cfblk6/1 -> cyemi_76/1

== system sampleModel2403_pp_difftest/cfblk114 ==
  cfblk1 : Inport
  cfblk8 : Inport  Port=2
  cfblk9 : Inport  Port=3
  Action Port : ActionPort  ActionType=then
  cfblk11 : Delay
  cfblk12 : DataTypeConversion  OutDataTypeStr=double
  cfblk3 : DiscreteZeroPole  Poles=[0 0.5]  Gain=1  SampleTime=-1
  cfblk4 : Delay  ShowEnablePort=on
      settings: InputPortMap=u0,e6
  cfblk5 : Delay  ShowEnablePort=on
      settings: InputPortMap=u0,e6
  cfblk6 : DiscreteTransferFcn
  cfblk7 : simulink/Discrete/Transfer Fcn Real Zero  ZeroZ=0.75  ICPrevInput=0.0  DoSatur=off
      settings: SourceProductName=Simulink  SourceProductBaseCode=SL
  cyemi_{80,82..88} (8 alike) : DataTypeConversion  OutDataTypeStr=double
  cyemi_81 : DataTypeConversion  OutDataTypeStr=uint16
  cfblk2 : Outport
  cfblk10 : Outport  Port=2
  wires:
  cfblk4/1 -> cfblk2/1
  cfblk9/1 -> cfblk10/1
  cfblk1/1 -> cyemi_84/1, cyemi_88/1
  cyemi_80/1 -> cfblk11/1
  cfblk6/1 -> cyemi_80/1
  cyemi_81/1 -> cfblk12/1
  cfblk8/1 -> cyemi_81/1
  cyemi_82/1 -> cfblk3/1
  cfblk12/1 -> cyemi_82/1
  cyemi_83/1 -> cfblk4/1
  cfblk7/1 -> cyemi_83/1
  cyemi_84/1 -> cfblk4/2
  cyemi_85/1 -> cfblk5/1
  cfblk11/1 -> cyemi_85/1
  cyemi_86/1 -> cfblk5/2
  cfblk3/1 -> cyemi_86/1
  cyemi_87/1 -> cfblk6/1
  cfblk5/1 -> cyemi_87/1
  cyemi_88/1 -> cfblk7/1

== system sampleModel2403_pp_difftest/cfblk115 ==
  cfblk1 : Inport
  cfblk8 : Inport  Port=2
  Action Port : ActionPort  ActionType=else
  cfblk3 : DiscreteIntegrator  SampleTime=-1  OutDataTypeStr=double  ICPrevOutput=DiscIntNeverNeededParam  ICPrevScaledInput=DiscIntNeverNeededParam
  cfblk4 : DiscreteTransferFcn
  cfblk5 : Delay  DelayLengthSource=Input port
      settings: InputPortMap=u0,p1
  cfblk6 : DiscreteTransferFcn
  cfblk7 : UnitDelay  SampleTime=-1
  cyemi_{91..96} (6 alike) : DataTypeConversion  OutDataTypeStr=double
  cfblk2 : Outport
  wires:
  cfblk4/1 -> cfblk2/1
  cyemi_91/1 -> cfblk3/1
  cfblk1/1 -> cyemi_91/1
  cyemi_92/1 -> cfblk4/1
  cfblk7/1 -> cyemi_92/1
  cyemi_93/1 -> cfblk5/1
  cfblk8/1 -> cyemi_93/1
  cyemi_94/1 -> cfblk5/2
  cfblk3/1 -> cyemi_94/1
  cyemi_95/1 -> cfblk6/1
  cfblk5/1 -> cyemi_95/1
  cyemi_96/1 -> cfblk7/1
  cfblk6/1 -> cyemi_96/1

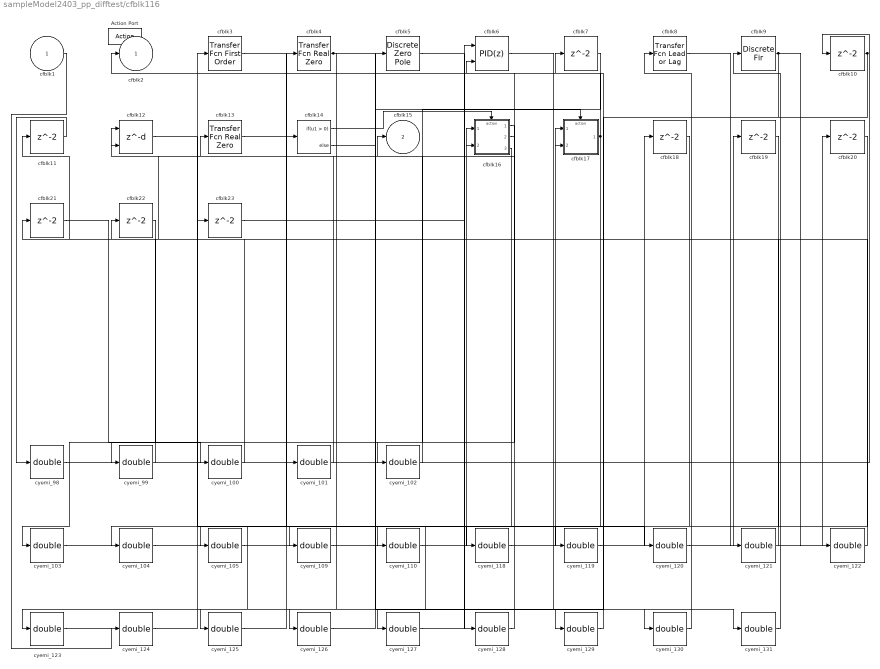
== system sampleModel2403_pp_difftest/cfblk116 ==
  cfblk1 : Inport
  Action Port : ActionPort  ActionType=then
  cfblk{7,10..11,18..23} (9 alike) : Delay
  cfblk12 : Delay  DelayLengthSource=Input port
      settings: InputPortMap=u0,p1
  cfblk13 : simulink/Discrete/Transfer Fcn Real Zero  ZeroZ=0.75  ICPrevInput=0.0  DoSatur=off
      settings: SourceProductName=Simulink  SourceProductBaseCode=SL
  cfblk14 : If  SampleTime=1
  cfblk16 : Subsystem  TreatAsAtomicUnit=on
  cfblk17 : Subsystem  TreatAsAtomicUnit=on
  cfblk3 : simulink/Discrete/Transfer Fcn First Order  PoleZ=0.95  ICPrevOutput=0.0  DoSatur=off
      settings: SourceProductName=Simulink
  cfblk4 : simulink/Discrete/Transfer Fcn Real Zero  ZeroZ=0.75  ICPrevInput=0.0  DoSatur=off
      settings: SourceProductName=Simulink  SourceProductBaseCode=SL
  cfblk5 : DiscreteZeroPole  Poles=[0 0.5]  Gain=1  SampleTime=-1
  cfblk6 : simulink/Continuous/PID Controller (2DOF)  Controller=PID  TimeDomain=Discrete-time  SampleTime=-1  IntegratorMethod=Forward Euler  FilterMethod=Forward Euler  Form=Parallel  UseFilter=on  ControllerParametersSource=internal  P=1  I=1  D=0  N=100  b=1  c=1  InitialConditionSource=internal  InitialConditionForIntegrator=0  InitialConditionForFilter=0  ExternalReset=none  LimitOutput=off  UpperSaturationLimit=inf  LowerSaturationLimit=-inf  LinearizeAsGain=off  AntiWindupMode=none  Kb=1  TrackingMode=off  Kt=1  PParamMin=[]  PParamMax=[]  IParamMin=[]  IParamMax=[]  DParamMin=[]  DParamMax=[]  NParamMin=[]  NParamMax=[]  bParamMin=[]  bParamMax=[]  cParamMin=[]  cParamMax=[]  KbParamMin=[]  KbParamMax=[]  KtParamMin=[]  KtParamMax=[]  POutMin=[]  POutMax=[]  IOutMin=[]  IOutMax=[]  DOutMin=[]  DOutMax=[]  NOutMin=[]  NOutMax=[]  bOutMin=[]  bOutMax=[]  cOutMin=[]  cOutMax=[]  KbOutMin=[]  KbOutMax=[]  KtOutMin=[]  KtOutMax=[]  IntegratorOutMin=[]  IntegratorOutMax=[]  FilterOutMin=[]  FilterOutMax=[]  SumOutMin=[]  SumOutMax=[]  Sum1OutMin=[]  Sum1OutMax=[]  Sum2OutMin=[]  Sum2OutMax=[]  Sum3OutMin=[]  Sum3OutMax=[]  SumI1OutMin=[]  SumI1OutMax=[]  SumI2OutMin=[]  SumI2OutMax=[]  SumI3OutMin=[]  SumI3OutMax=[]  SumDOutMin=[]  SumDOutMax=[]  SaturationOutMin=[]  SaturationOutMax=[]  IntegratorContinuousStateAttributes=''  IntegratorStateMustResolveToSignalObject=off  IntegratorRTWStateStorageClass=Auto  FilterContinuousStateAttributes=''  FilterStateMustResolveToSignalObject=off  FilterRTWStateStorageClass=Auto  DifferentiatorICPrevScaledInput=0  DifferentiatorOutMin=[]  DifferentiatorOutMax=[]  FilterDiffOutCoefMin=[]  FilterDiffOutCoefMax=[]  SumDenOutMin=[]  SumDenOutMax=[]  SumNumOutMin=[]  SumNumOutMax=[]  ReciprocalOutMin=[]  ReciprocalOutMax=[]  DivideOutMin=[]  DivideOutMax=[]  TunerSelectOption=Transfer Function Based (PID Tuner App)
  cfblk8 : simulink/Discrete/Transfer Fcn Lead or Lag  PoleZ=0.95  ZeroZ=0.75  ICPrevOutput=0.0  ICPrevInput=0.0  DoSatur=off
      settings: SourceProductName=Simulink  SourceProductBaseCode=SL
  cfblk9 : DiscreteFir
  cyemi_{98..105,109..110,118..131} (24 alike) : DataTypeConversion  OutDataTypeStr=double
  cfblk2 : Outport
  cfblk15 : Outport  Port=2
  wires:
  cfblk9/1 -> cyemi_122/1, cyemi_123/1
  cfblk17/1(cfblk2) -> cfblk2/1, cyemi_127/1
  cfblk4/1 -> cyemi_126/1, cyemi_130/1
  cfblk10/1 -> cyemi_118/1, cyemi_119/1
  cfblk16/2(cfblk7) -> cfblk15/1
  cfblk14/1 -> cfblk16/Action
  cfblk14/2 -> cfblk17/Action
  cyemi_98/1 -> cfblk10/1
  cfblk11/1 -> cyemi_98/1
  cyemi_99/1 -> cfblk11/1
  cfblk16/1(cfblk2) -> cyemi_99/1
  cyemi_100/1 -> cfblk12/1
  cfblk21/1 -> cyemi_100/1
  cyemi_101/1 -> cfblk12/2
  cfblk3/1 -> cyemi_101/1
  cyemi_102/1 -> cfblk13/1
  cfblk7/1 -> cyemi_102/1
  cyemi_103/1 -> cfblk14/1
  cfblk22/1 -> cyemi_103/1
  cyemi_104/1 -> cfblk16/1(cfblk1)
  cfblk18/1 -> cyemi_104/1
  cyemi_105/1 -> cfblk16/2(cfblk6)
  cfblk20/1 -> cyemi_105/1
  cyemi_109/1 -> cfblk17/1(cfblk1)
  cfblk12/1 -> cyemi_109/1
  cyemi_110/1 -> cfblk17/2(cfblk8)
  cfblk19/1 -> cyemi_110/1
  cyemi_118/1 -> cfblk18/1
  cyemi_119/1 -> cfblk19/1
  cyemi_120/1 -> cfblk20/1
  cfblk13/1 -> cyemi_120/1
  cyemi_121/1 -> cfblk21/1
  cfblk8/1 -> cyemi_121/1
  cyemi_122/1 -> cfblk22/1
  cyemi_123/1 -> cfblk23/1
  cyemi_124/1 -> cfblk3/1
  cfblk1/1 -> cyemi_124/1
  cyemi_125/1 -> cfblk4/1
  cfblk16/3(cfblk8) -> cyemi_125/1
  cyemi_126/1 -> cfblk5/1
  cyemi_127/1 -> cfblk6/1
  cyemi_128/1 -> cfblk6/2
  cfblk23/1 -> cyemi_128/1
  cyemi_129/1 -> cfblk7/1
  cfblk5/1 -> cyemi_129/1
  cyemi_130/1 -> cfblk8/1
  cyemi_131/1 -> cfblk9/1
  cfblk6/1 -> cyemi_131/1

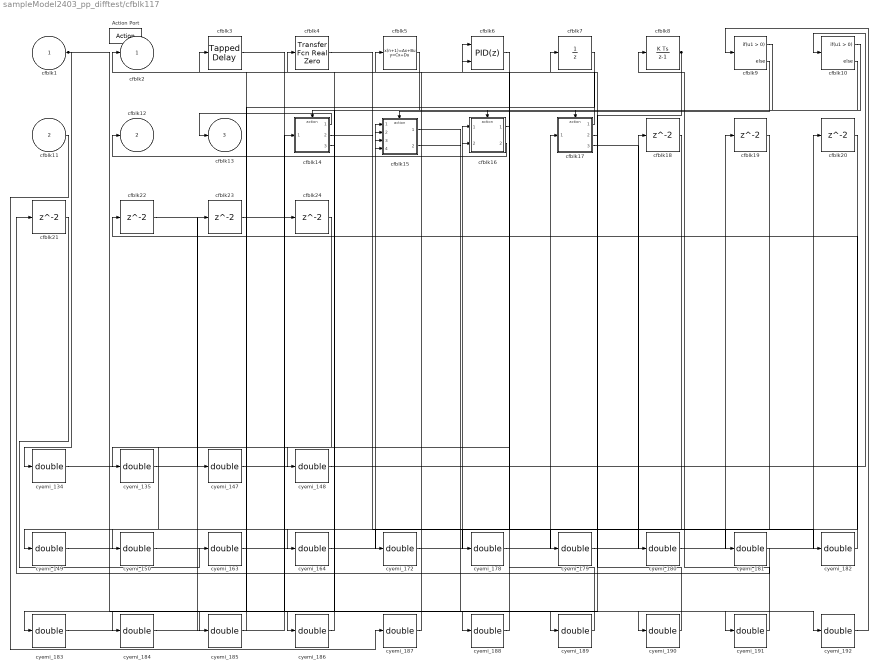
== system sampleModel2403_pp_difftest/cfblk117 ==
  cfblk1 : Inport
  cfblk11 : Inport  Port=2
  Action Port : ActionPort  ActionType=else
  cfblk10 : If  SampleTime=1
  cfblk14 : Subsystem  TreatAsAtomicUnit=on
  cfblk15 : Subsystem  TreatAsAtomicUnit=on
  cfblk16 : Subsystem  TreatAsAtomicUnit=on
  cfblk17 : Subsystem  TreatAsAtomicUnit=on
  cfblk{18..24} (7 alike) : Delay
  cfblk3 : simulink/Discrete/Tapped Delay  vinit=0.0  samptime=-1  NumDelays=1  DelayOrder=Oldest  includeCurrent=off
  cfblk4 : simulink/Discrete/Transfer Fcn Real Zero  ZeroZ=0.75  ICPrevInput=0.0  DoSatur=off
      settings: SourceProductName=Simulink  SourceProductBaseCode=SL
  cfblk5 : DiscreteStateSpace  SampleTime=-1
  cfblk6 : simulink/Continuous/PID Controller (2DOF)  Controller=PID  TimeDomain=Discrete-time  SampleTime=-1  IntegratorMethod=Forward Euler  FilterMethod=Forward Euler  Form=Parallel  UseFilter=on  ControllerParametersSource=internal  P=1  I=1  D=0  N=100  b=1  c=1  InitialConditionSource=internal  InitialConditionForIntegrator=0  InitialConditionForFilter=0  ExternalReset=none  LimitOutput=off  UpperSaturationLimit=inf  LowerSaturationLimit=-inf  LinearizeAsGain=off  AntiWindupMode=none  Kb=1  TrackingMode=off  Kt=1  PParamMin=[]  PParamMax=[]  IParamMin=[]  IParamMax=[]  DParamMin=[]  DParamMax=[]  NParamMin=[]  NParamMax=[]  bParamMin=[]  bParamMax=[]  cParamMin=[]  cParamMax=[]  KbParamMin=[]  KbParamMax=[]  KtParamMin=[]  KtParamMax=[]  POutMin=[]  POutMax=[]  IOutMin=[]  IOutMax=[]  DOutMin=[]  DOutMax=[]  NOutMin=[]  NOutMax=[]  bOutMin=[]  bOutMax=[]  cOutMin=[]  cOutMax=[]  KbOutMin=[]  KbOutMax=[]  KtOutMin=[]  KtOutMax=[]  IntegratorOutMin=[]  IntegratorOutMax=[]  FilterOutMin=[]  FilterOutMax=[]  SumOutMin=[]  SumOutMax=[]  Sum1OutMin=[]  Sum1OutMax=[]  Sum2OutMin=[]  Sum2OutMax=[]  Sum3OutMin=[]  Sum3OutMax=[]  SumI1OutMin=[]  SumI1OutMax=[]  SumI2OutMin=[]  SumI2OutMax=[]  SumI3OutMin=[]  SumI3OutMax=[]  SumDOutMin=[]  SumDOutMax=[]  SaturationOutMin=[]  SaturationOutMax=[]  IntegratorContinuousStateAttributes=''  IntegratorStateMustResolveToSignalObject=off  IntegratorRTWStateStorageClass=Auto  FilterContinuousStateAttributes=''  FilterStateMustResolveToSignalObject=off  FilterRTWStateStorageClass=Auto  DifferentiatorICPrevScaledInput=0  DifferentiatorOutMin=[]  DifferentiatorOutMax=[]  FilterDiffOutCoefMin=[]  FilterDiffOutCoefMax=[]  SumDenOutMin=[]  SumDenOutMax=[]  SumNumOutMin=[]  SumNumOutMax=[]  ReciprocalOutMin=[]  ReciprocalOutMax=[]  DivideOutMin=[]  DivideOutMax=[]  TunerSelectOption=Transfer Function Based (PID Tuner App)
  cfblk7 : UnitDelay  SampleTime=-1
  cfblk8 : DiscreteIntegrator  SampleTime=-1  OutDataTypeStr=double  ICPrevOutput=DiscIntNeverNeededParam  ICPrevScaledInput=DiscIntNeverNeededParam
  cfblk9 : If  SampleTime=1
  cyemi_{134..135,147..150,163..164,172,178..192} (24 alike) : DataTypeConversion  OutDataTypeStr=double
  cfblk2 : Outport
  cfblk12 : Outport  Port=2
  cfblk13 : Outport  Port=3
  wires:
  cfblk17/1(cfblk2) -> cfblk2/1
  cfblk1/1 -> cyemi_134/1, cyemi_189/1
  cfblk14/1(cfblk2) -> cfblk13/1
  cfblk8/1 -> cyemi_183/1, cyemi_184/1
  cfblk16/2(cfblk9) -> cfblk12/1
  cfblk9/1 -> cfblk14/Action
  cfblk9/2 -> cfblk15/Action
  cfblk10/1 -> cfblk16/Action
  cfblk10/2 -> cfblk17/Action
  cyemi_134/1 -> cfblk10/1
  cyemi_135/1 -> cfblk14/1(cfblk1)
  cfblk5/1 -> cyemi_135/1
  cyemi_147/1 -> cfblk15/1(cfblk1)
  cfblk22/1 -> cyemi_147/1
  cyemi_148/1 -> cfblk15/2(cfblk14)
  cfblk16/1(cfblk2) -> cyemi_148/1
  cyemi_149/1 -> cfblk15/3(cfblk15)
  cfblk20/1 -> cyemi_149/1
  cyemi_150/1 -> cfblk15/4(cfblk16)
  cfblk24/1 -> cyemi_150/1
  cyemi_163/1 -> cfblk16/1(cfblk1)
  cfblk21/1 -> cyemi_163/1
  cyemi_164/1 -> cfblk16/2(cfblk8)
  cfblk19/1 -> cyemi_164/1
  cyemi_172/1 -> cfblk17/1(cfblk1)
  cfblk18/1 -> cyemi_172/1
  cyemi_178/1 -> cfblk18/1
  cfblk6/1 -> cyemi_178/1
  cyemi_179/1 -> cfblk19/1
  cfblk17/2(cfblk7) -> cyemi_179/1
  cyemi_180/1 -> cfblk20/1
  cfblk17/3(cfblk8) -> cyemi_180/1
  cyemi_181/1 -> cfblk21/1
  cfblk14/2(cfblk11) -> cyemi_181/1
  cyemi_182/1 -> cfblk22/1
  cfblk4/1 -> cyemi_182/1
  cyemi_183/1 -> cfblk23/1
  cyemi_184/1 -> cfblk24/1
  cyemi_185/1 -> cfblk3/1
  cfblk7/1 -> cyemi_185/1
  cyemi_186/1 -> cfblk4/1
  cfblk14/3(cfblk12) -> cyemi_186/1
  cyemi_187/1 -> cfblk5/1
  cfblk11/1 -> cyemi_187/1
  cyemi_188/1 -> cfblk6/1
  cfblk3/1 -> cyemi_188/1
  cyemi_189/1 -> cfblk6/2
  cyemi_190/1 -> cfblk7/1
  cfblk15/1(cfblk2) -> cyemi_190/1
  cyemi_191/1 -> cfblk8/1
  cfblk15/2(cfblk17) -> cyemi_191/1
  cyemi_192/1 -> cfblk9/1
  cfblk23/1 -> cyemi_192/1

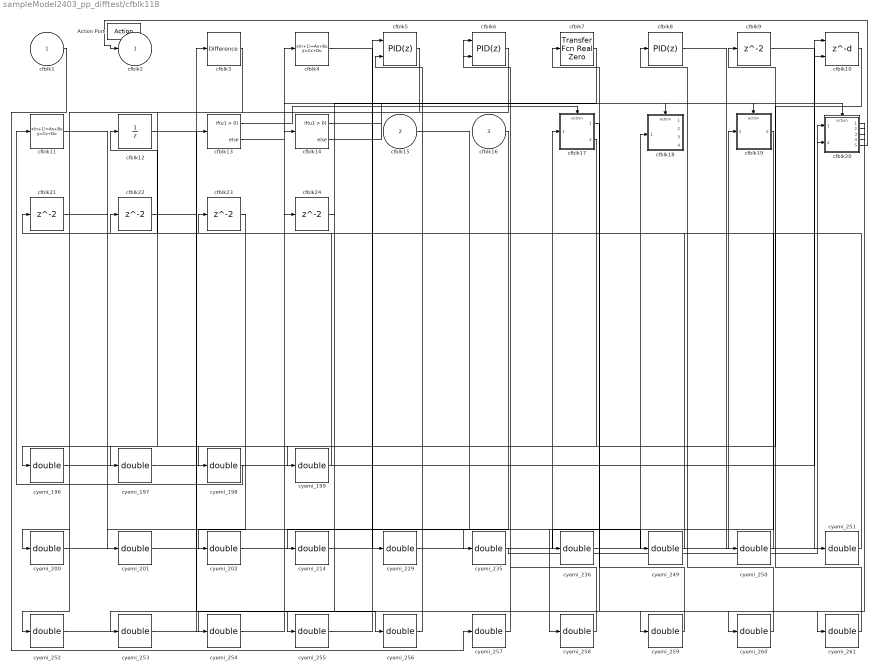
== system sampleModel2403_pp_difftest/cfblk118 ==
  cfblk1 : Inport
  cfblk15 : Inport  Port=2
  cfblk16 : Inport  Port=3
  Action Port : ActionPort  ActionType=then
  cfblk10 : Delay  DelayLengthSource=Input port
      settings: InputPortMap=u0,p1
  cfblk11 : DiscreteStateSpace  SampleTime=-1
  cfblk12 : UnitDelay  SampleTime=-1
  cfblk13 : If  SampleTime=1
  cfblk14 : If  SampleTime=1
  cfblk17 : Subsystem  TreatAsAtomicUnit=on
  cfblk18 : Subsystem  TreatAsAtomicUnit=on
  cfblk19 : Subsystem  TreatAsAtomicUnit=on
  cfblk20 : Subsystem  TreatAsAtomicUnit=on
  cfblk{9,21..24} (5 alike) : Delay
  cfblk3 : simulink/Discrete/Difference  ICPrevInput=0.0  OutMin=[]  OutMax=[]  OutDataTypeStr=double  OutputDataTypeScalingMode=double  OutDataType=fixdt(1, 16)  OutScaling=2^-10  DoSatur=off
  cfblk4 : DiscreteStateSpace  SampleTime=-1
  cfblk5 : simulink/Continuous/PID Controller (2DOF)  Controller=PID  TimeDomain=Discrete-time  SampleTime=-1  IntegratorMethod=Forward Euler  FilterMethod=Forward Euler  Form=Parallel  UseFilter=on  ControllerParametersSource=internal  P=1  I=1  D=0  N=100  b=1  c=1  InitialConditionSource=internal  InitialConditionForIntegrator=0  InitialConditionForFilter=0  ExternalReset=none  LimitOutput=off  UpperSaturationLimit=inf  LowerSaturationLimit=-inf  LinearizeAsGain=off  AntiWindupMode=none  Kb=1  TrackingMode=off  Kt=1  PParamMin=[]  PParamMax=[]  IParamMin=[]  IParamMax=[]  DParamMin=[]  DParamMax=[]  NParamMin=[]  NParamMax=[]  bParamMin=[]  bParamMax=[]  cParamMin=[]  cParamMax=[]  KbParamMin=[]  KbParamMax=[]  KtParamMin=[]  KtParamMax=[]  POutMin=[]  POutMax=[]  IOutMin=[]  IOutMax=[]  DOutMin=[]  DOutMax=[]  NOutMin=[]  NOutMax=[]  bOutMin=[]  bOutMax=[]  cOutMin=[]  cOutMax=[]  KbOutMin=[]  KbOutMax=[]  KtOutMin=[]  KtOutMax=[]  IntegratorOutMin=[]  IntegratorOutMax=[]  FilterOutMin=[]  FilterOutMax=[]  SumOutMin=[]  SumOutMax=[]  Sum1OutMin=[]  Sum1OutMax=[]  Sum2OutMin=[]  Sum2OutMax=[]  Sum3OutMin=[]  Sum3OutMax=[]  SumI1OutMin=[]  SumI1OutMax=[]  SumI2OutMin=[]  SumI2OutMax=[]  SumI3OutMin=[]  SumI3OutMax=[]  SumDOutMin=[]  SumDOutMax=[]  SaturationOutMin=[]  SaturationOutMax=[]  IntegratorContinuousStateAttributes=''  IntegratorStateMustResolveToSignalObject=off  IntegratorRTWStateStorageClass=Auto  FilterContinuousStateAttributes=''  FilterStateMustResolveToSignalObject=off  FilterRTWStateStorageClass=Auto  DifferentiatorICPrevScaledInput=0  DifferentiatorOutMin=[]  DifferentiatorOutMax=[]  FilterDiffOutCoefMin=[]  FilterDiffOutCoefMax=[]  SumDenOutMin=[]  SumDenOutMax=[]  SumNumOutMin=[]  SumNumOutMax=[]  ReciprocalOutMin=[]  ReciprocalOutMax=[]  DivideOutMin=[]  DivideOutMax=[]  TunerSelectOption=Transfer Function Based (PID Tuner App)
  cfblk6 : simulink/Continuous/PID Controller (2DOF)  Controller=PID  TimeDomain=Discrete-time  SampleTime=-1  IntegratorMethod=Forward Euler  FilterMethod=Forward Euler  Form=Parallel  UseFilter=on  ControllerParametersSource=internal  P=1  I=1  D=0  N=100  b=1  c=1  InitialConditionSource=internal  InitialConditionForIntegrator=0  InitialConditionForFilter=0  ExternalReset=none  LimitOutput=off  UpperSaturationLimit=inf  LowerSaturationLimit=-inf  LinearizeAsGain=off  AntiWindupMode=none  Kb=1  TrackingMode=off  Kt=1  PParamMin=[]  PParamMax=[]  IParamMin=[]  IParamMax=[]  DParamMin=[]  DParamMax=[]  NParamMin=[]  NParamMax=[]  bParamMin=[]  bParamMax=[]  cParamMin=[]  cParamMax=[]  KbParamMin=[]  KbParamMax=[]  KtParamMin=[]  KtParamMax=[]  POutMin=[]  POutMax=[]  IOutMin=[]  IOutMax=[]  DOutMin=[]  DOutMax=[]  NOutMin=[]  NOutMax=[]  bOutMin=[]  bOutMax=[]  cOutMin=[]  cOutMax=[]  KbOutMin=[]  KbOutMax=[]  KtOutMin=[]  KtOutMax=[]  IntegratorOutMin=[]  IntegratorOutMax=[]  FilterOutMin=[]  FilterOutMax=[]  SumOutMin=[]  SumOutMax=[]  Sum1OutMin=[]  Sum1OutMax=[]  Sum2OutMin=[]  Sum2OutMax=[]  Sum3OutMin=[]  Sum3OutMax=[]  SumI1OutMin=[]  SumI1OutMax=[]  SumI2OutMin=[]  SumI2OutMax=[]  SumI3OutMin=[]  SumI3OutMax=[]  SumDOutMin=[]  SumDOutMax=[]  SaturationOutMin=[]  SaturationOutMax=[]  IntegratorContinuousStateAttributes=''  IntegratorStateMustResolveToSignalObject=off  IntegratorRTWStateStorageClass=Auto  FilterContinuousStateAttributes=''  FilterStateMustResolveToSignalObject=off  FilterRTWStateStorageClass=Auto  DifferentiatorICPrevScaledInput=0  DifferentiatorOutMin=[]  DifferentiatorOutMax=[]  FilterDiffOutCoefMin=[]  FilterDiffOutCoefMax=[]  SumDenOutMin=[]  SumDenOutMax=[]  SumNumOutMin=[]  SumNumOutMax=[]  ReciprocalOutMin=[]  ReciprocalOutMax=[]  DivideOutMin=[]  DivideOutMax=[]  TunerSelectOption=Transfer Function Based (PID Tuner App)
  cfblk7 : simulink/Discrete/Transfer Fcn Real Zero  ZeroZ=0.75  ICPrevInput=0.0  DoSatur=off
      settings: SourceProductName=Simulink  SourceProductBaseCode=SL
  cfblk8 : simulink/Continuous/PID Controller  Controller=PID  TimeDomain=Discrete-time  SampleTime=-1  IntegratorMethod=Forward Euler  FilterMethod=Forward Euler  Form=Parallel  UseFilter=on  ControllerParametersSource=internal  P=1  I=1  D=0  N=100  InitialConditionSource=internal  InitialConditionForIntegrator=0  InitialConditionForFilter=0  ExternalReset=none  LimitOutput=off  UpperSaturationLimit=inf  LowerSaturationLimit=-inf  LinearizeAsGain=off  AntiWindupMode=none  Kb=1  TrackingMode=off  Kt=1  PParamMin=[]  PParamMax=[]  IParamMin=[]  IParamMax=[]  DParamMin=[]  DParamMax=[]  NParamMin=[]  NParamMax=[]  KbParamMin=[]  KbParamMax=[]  KtParamMin=[]  KtParamMax=[]  POutMin=[]  POutMax=[]  IOutMin=[]  IOutMax=[]  DOutMin=[]  DOutMax=[]  NOutMin=[]  NOutMax=[]  KbOutMin=[]  KbOutMax=[]  KtOutMin=[]  KtOutMax=[]  IntegratorOutMin=[]  IntegratorOutMax=[]  FilterOutMin=[]  FilterOutMax=[]  SumOutMin=[]  SumOutMax=[]  SumI1OutMin=[]  SumI1OutMax=[]  SumI2OutMin=[]  SumI2OutMax=[]  SumI3OutMin=[]  SumI3OutMax=[]  SumDOutMin=[]  SumDOutMax=[]  SaturationOutMin=[]  SaturationOutMax=[]  IntegratorContinuousStateAttributes=''  IntegratorStateMustResolveToSignalObject=off  IntegratorRTWStateStorageClass=Auto  FilterContinuousStateAttributes=''  FilterStateMustResolveToSignalObject=off  FilterRTWStateStorageClass=Auto  DifferentiatorICPrevScaledInput=0  DifferentiatorOutMin=[]  DifferentiatorOutMax=[]  FilterDiffOutCoefMin=[]  FilterDiffOutCoefMax=[]  SumDenOutMin=[]  SumDenOutMax=[]  SumNumOutMin=[]  SumNumOutMax=[]  ReciprocalOutMin=[]  ReciprocalOutMax=[]  DivideOutMin=[]  DivideOutMax=[]  TunerSelectOption=Transfer Function Based (PID Tuner App)
  cyemi_{196..202,214,229,235..236,249..261} (24 alike) : DataTypeConversion  OutDataTypeStr=double
  cfblk2 : Outport
  wires:
  cfblk20/5(cfblk17) -> cfblk2/1
  cfblk13/1 -> cfblk17/Action
  cfblk13/2 -> cfblk18/Action
  cfblk14/1 -> cfblk19/Action
  cfblk14/2 -> cfblk20/Action
  cyemi_196/1 -> cfblk10/1
  cfblk17/2(cfblk11) -> cyemi_196/1
  cyemi_197/1 -> cfblk10/2
  cfblk3/1 -> cyemi_197/1
  cyemi_198/1 -> cfblk11/1
  cfblk10/1 -> cyemi_198/1
  cyemi_199/1 -> cfblk12/1
  cfblk7/1 -> cyemi_199/1
  cyemi_200/1 -> cfblk13/1
  cfblk6/1 -> cyemi_200/1
  cyemi_201/1 -> cfblk14/1
  cfblk21/1 -> cyemi_201/1
  cyemi_202/1 -> cfblk17/1(cfblk1)
  cfblk23/1 -> cyemi_202/1
  cyemi_214/1 -> cfblk18/1(cfblk1)
  cfblk24/1 -> cyemi_214/1
  cyemi_229/1 -> cfblk19/1(cfblk1)
  cfblk4/1 -> cyemi_229/1
  cyemi_235/1 -> cfblk20/1(cfblk1)
  cfblk22/1 -> cyemi_235/1
  cyemi_236/1 -> cfblk20/2(cfblk13)
  cfblk19/1(cfblk2) -> cyemi_236/1
  cyemi_249/1 -> cfblk21/1
  cfblk11/1 -> cyemi_249/1
  cyemi_250/1 -> cfblk22/1
  cfblk8/1 -> cyemi_250/1
  cyemi_251/1 -> cfblk23/1
  cfblk9/1 -> cyemi_251/1
  cyemi_252/1 -> cfblk24/1
  cfblk5/1 -> cyemi_252/1
  cyemi_253/1 -> cfblk3/1
  cfblk20/1(cfblk2) -> cyemi_253/1
  cyemi_254/1 -> cfblk4/1
  cfblk17/1(cfblk2) -> cyemi_254/1
  cyemi_255/1 -> cfblk5/1
  cfblk16/1 -> cyemi_255/1
  cyemi_256/1 -> cfblk5/2
  cfblk12/1 -> cyemi_256/1
  cyemi_257/1 -> cfblk6/1
  cfblk1/1 -> cyemi_257/1
  cyemi_258/1 -> cfblk6/2
  cfblk15/1 -> cyemi_258/1
  cyemi_259/1 -> cfblk7/1
  cfblk20/4(cfblk16) -> cyemi_259/1
  cyemi_260/1 -> cfblk8/1
  cfblk20/2(cfblk14) -> cyemi_260/1
  cyemi_261/1 -> cfblk9/1
  cfblk20/3(cfblk15) -> cyemi_261/1
